simulink model "Battery_v4"  (R2024b)
settings: Solver=VariableStepAuto  StartTime=0.0  StopTime=inf  RelTol=1e-3
settings Model: Creator=miche  LastModifiedBy=miche

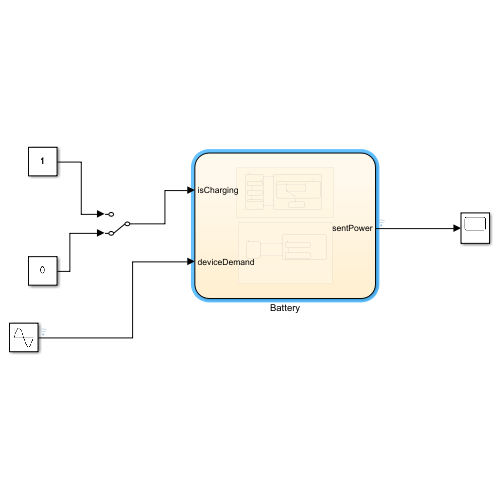
[thumbnail: Simulink's stored preview of the top-level diagram]
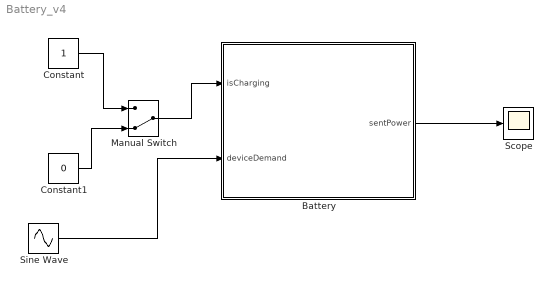
== system Battery_v4 ==
  Battery : Stateflow chart  TreatAsAtomicUnit=on
  Constant : Constant  SampleTime=0.5
  Constant1 : Constant  Value=0  SampleTime=0.5
  Manual Switch : ManualSwitch  CurrentSetting=0
  Scope : Scope
  Sine Wave : Sin  Amplitude=2.5  Bias=2.5  Phase=-pi/4  SampleTime=0
  wires:
  Constant/1 -> Manual Switch/1
  Constant1/1 -> Manual Switch/2
  Manual Switch/1 -> Battery/1(isCharging)
  Battery/1(sentPower) -> Scope/1
  Sine Wave/1 -> Battery/2(deviceDemand)

== stateflow chart Battery_v4/Battery ==
  state MainBattery [parallel]
    settings: executionOrder=1
    state Charge
      entry:
      sentPower = 0;
      send(toggleOff, EmergencyBattery)
      state FastCharge
        during:
        mainCharge = mainCharge+4;
      state SlowChart
        during:
        mainCharge = mainCharge +1
      state Full
      (default) -> FastCharge
      FastCharge -> SlowChart : [mainCharge > 80]
      SlowChart -> Full : [mainCharge == 100]
    state Discharge
      state Powered
        MainBattery.Discharge.Powered -> (junction 19) [order 1]
        (junction 19) -> (junction 20) [order 1] : [deviceDemand>maxPower]
        (junction 19) -> (junction 24) [order 2] : {sentPower = deviceDemand;}
        (junction 20) -> (junction 21) : {sentPower = maxPower;}
        (junction 21) -> (junction 24)
        (junction 24) -> (junction 27) : {mainCharge = mainCharge- sentPower; }
      state Empty
        entry:
        sentPower = 0;
        send(toggleOn, EmergencyBattery)
      (default) -> MainBattery.Discharge.Powered
      MainBattery.Discharge.Powered -> MainBattery.Discharge.Empty [order 1] : [mainCharge<=3]
    (default) -> Charge
    Charge -> MainBattery.Discharge : [~isCharging]
    MainBattery.Discharge -> Charge : [isCharging]
  state EmergencyBattery [parallel]
    settings: executionOrder=2
    state Discharge
      state Powered
        during:
        emergencyCharge = emergencyCharge - 0.01;
      state Empty
      (default) -> EmergencyBattery.Discharge.Powered
      EmergencyBattery.Discharge.Powered -> EmergencyBattery.Discharge.Empty : [emergencyCharge<=0.01]
    state Standby
    (default) -> Standby
    Standby -> EmergencyBattery.Discharge : toggleOn
    EmergencyBattery.Discharge -> Standby : toggleOff
  data: isCharging input; sentPower output; maxPower local =3.5; deviceDemand input; mainCharge local =50; emergencyCharge local =3
  events: toggleOn local FUNCTION_CALL_EVENT; toggleOff local FUNCTION_CALL_EVENT
